simulink model "ALL_JP360_DBW_V6_5_1103"  (R2022a)
settings: Solver=FixedStepAuto  StartTime=0.0  StopTime=inf  FixedStep=0.01  RelTol=1e-3  EnableMultiTasking=on
model workspace (MAT data in the model file):
  g = 9.8
undefined symbols (not defined in the file or in its folder): canChannel, delta_v_p, IPM_Line_C0, IPM_Line_C1, IPM_Line_C2, IPM_Line_C3, M, M_p, MRR_ObjDistX, MRR_ObjDistY, MRR_ObjFusionCamID, MRR_ObjFusionSig, MRR_ObjID, MRR_ObjRelVelX, MRR_ObjRelVelY, MRR_ObjType, MRR_ObjUpdFlg, none, obj_vaild, untracktime, V, videoinput
libraries: canfdmsglib x230, canfdlib x76, slpidlib x24, simulink x18, dspstat3 x14, ctrlSharedLib x1, simulink_extras x1, imaqlib x1, realtime_pacer_lib x1, dspvision x1, visionsinks x1
(part 15 of 55)

== system ALL_JP360_DBW_V6_5_1103/MsgFromCAN/CCAN_GW_MsgFromCAN/CCAN_GW_SRR_FL_0x27B ==
  CCAN_GW_SRR_FL_0x27BFromInData : Inport  OutDataTypeStr=Bus:CAN_FD_MESSAGE_BUS
  Bus Creator : BusCreator  Inputs=8  OutDataTypeStr=Bus:CCAN_GW_SRR_FL_0x27B  NonVirtualBus=on
  CAN FD Unpack : canfdmsglib/CAN FD Unpack  CANdbFile=HiFire_JPT360_CCAN_Matrix_CAN_V1.72_VP_ADCU.dbc  MsgList=(none)  MsgName=SRR_FL_0x27B  ProtocolMode=CAN FD  MsgIDType=Standard (11-bit identifier)  MsgIdentifier=635  MsgLength=8  SignalInfo={'BSD_FCTA_Active','0','2','BE','unsigned','Standard','0','1','0','0','3';'BSD_FCTA_State','7','1','BE','unsigned','Standard','0','1','0','0','1';'BSD_FCTA_display','12','4','BE','unsigned','Standard','0','1','0','0','15';'Checksum_0x27B','56','8','BE','unsigned','Standard','0','1','0','0','255';'FCTA_OFFTelltale','6','1','BE','unsigned','Standard','0','1','0','0','1';'FCTA_warningReqLeft','4','2','BE','unsigned','Standard','0','1','0','0','3';'FCTA_warningReqRight','2','2','BE','unsigned','Standard','0','1','0','0','3';'RollingCounter_0x27B','48','4','BE','unsigned','Standard','0','1','0','0','15'}  IDPort=off  TimestampPort=off  ErrorPort=off  RemotePort=off  LengthPort=off  StatusPort=off  BRSPort=off  ESIPort=off  DLCPort=off  ApplyMinMax=off
      settings: SourceProductBaseCode=XP,ME,VN  DataFormat=CANdb specified signals
  Data Type Conversion{1,3,6..8} (5 alike) : DataTypeConversion  OutDataTypeStr=int8  SaturateOnIntegerOverflow=off  RndMeth=Floor
  Data Type Conversion2 : DataTypeConversion  OutDataTypeStr=boolean  SaturateOnIntegerOverflow=off  RndMeth=Floor
  Data Type Conversion4 : DataTypeConversion  OutDataTypeStr=uint8  SaturateOnIntegerOverflow=off  RndMeth=Floor
  Data Type Conversion5 : DataTypeConversion  OutDataTypeStr=boolean  SaturateOnIntegerOverflow=off  RndMeth=Floor
  CCAN_GW_SRR_FL_0x27BFromOutData : Outport  OutDataTypeStr=Bus:CCAN_GW_SRR_FL_0x27B
  wires:
  CAN FD Unpack/1 -> Data Type Conversion1/1
  CAN FD Unpack/2 -> Data Type Conversion2/1
  CAN FD Unpack/3 -> Data Type Conversion3/1
  CAN FD Unpack/4 -> Data Type Conversion4/1
  CAN FD Unpack/5 -> Data Type Conversion5/1
  CAN FD Unpack/6 -> Data Type Conversion6/1
  CAN FD Unpack/7 -> Data Type Conversion7/1
  CAN FD Unpack/8 -> Data Type Conversion8/1
  Data Type Conversion1/1 -> Bus Creator/1  "BSD_FCTA_Active"
  Data Type Conversion2/1 -> Bus Creator/2  "BSD_FCTA_State"
  Data Type Conversion3/1 -> Bus Creator/3  "BSD_FCTA_display"
  Data Type Conversion4/1 -> Bus Creator/4  "Checksum_0x27B"
  Data Type Conversion5/1 -> Bus Creator/5  "FCTA_OFFTelltale"
  Data Type Conversion6/1 -> Bus Creator/6  "FCTA_warningReqLeft"
  Data Type Conversion7/1 -> Bus Creator/7  "FCTA_warningReqRight"
  Data Type Conversion8/1 -> Bus Creator/8  "RollingCounter_0x27B"
  Bus Creator/1 -> CCAN_GW_SRR_FL_0x27BFromOutData/1  "CCAN_GW_SRR_FL_0x27BFromOutData"
  CCAN_GW_SRR_FL_0x27BFromInData/1 -> CAN FD Unpack/1  "CCAN_GW_SRR_FL_0x27BFromInData"

== system ALL_JP360_DBW_V6_5_1103/MsgFromCAN/CCAN_GW_MsgFromCAN/CCAN_GW_SRR_RL_0x27A ==
  CCAN_GW_SRR_RL_0x27AFromInData : Inport  OutDataTypeStr=Bus:CAN_FD_MESSAGE_BUS
  Bus Creator : BusCreator  Inputs=5  OutDataTypeStr=Bus:CCAN_GW_SRR_RL_0x27A  NonVirtualBus=on
  CAN FD Unpack : canfdmsglib/CAN FD Unpack  CANdbFile=HiFire_JPT360_CCAN_Matrix_CAN_V1.72_VP_ADCU.dbc  MsgList=(none)  MsgName=SRR_RL_0x27A  ProtocolMode=CAN FD  MsgIDType=Standard (11-bit identifier)  MsgIdentifier=634  MsgLength=8  SignalInfo={'BSD_RCTBTargetDeceleration','16','16','BE','unsigned','Standard','0','0.05','-16','-16','16';'BSD_RCTB_State','7','1','BE','unsigned','Standard','0','1','0','0','1';'BSD_RCTB_req','6','1','BE','unsigned','Standard','0','1','0','0','1';'Checksum_0x27A','56','8','BE','unsigned','Standard','0','1','0','0','255';'RollingCounter_0x27A','48','4','BE','unsigned','Standard','0','1','0','0','15'}  IDPort=off  TimestampPort=off  ErrorPort=off  RemotePort=off  LengthPort=off  StatusPort=off  BRSPort=off  ESIPort=off  DLCPort=off  ApplyMinMax=off
      settings: SourceProductBaseCode=XP,ME,VN  DataFormat=CANdb specified signals
  Data Type Conversion1 : DataTypeConversion  OutDataTypeStr=single  SaturateOnIntegerOverflow=off  RndMeth=Floor
  Data Type Conversion2 : DataTypeConversion  OutDataTypeStr=boolean  SaturateOnIntegerOverflow=off  RndMeth=Floor
  Data Type Conversion3 : DataTypeConversion  OutDataTypeStr=boolean  SaturateOnIntegerOverflow=off  RndMeth=Floor
  Data Type Conversion4 : DataTypeConversion  OutDataTypeStr=uint8  SaturateOnIntegerOverflow=off  RndMeth=Floor
  Data Type Conversion5 : DataTypeConversion  OutDataTypeStr=int8  SaturateOnIntegerOverflow=off  RndMeth=Floor
  CCAN_GW_SRR_RL_0x27AFromOutData : Outport  OutDataTypeStr=Bus:CCAN_GW_SRR_RL_0x27A
  wires:
  CAN FD Unpack/1 -> Data Type Conversion1/1
  CAN FD Unpack/2 -> Data Type Conversion2/1
  CAN FD Unpack/3 -> Data Type Conversion3/1
  CAN FD Unpack/4 -> Data Type Conversion4/1
  CAN FD Unpack/5 -> Data Type Conversion5/1
  Data Type Conversion1/1 -> Bus Creator/1  "BSD_RCTBTargetDeceleration"
  Data Type Conversion2/1 -> Bus Creator/2  "BSD_RCTB_State"
  Data Type Conversion3/1 -> Bus Creator/3  "BSD_RCTB_req"
  Data Type Conversion4/1 -> Bus Creator/4  "Checksum_0x27A"
  Data Type Conversion5/1 -> Bus Creator/5  "RollingCounter_0x27A"
  Bus Creator/1 -> CCAN_GW_SRR_RL_0x27AFromOutData/1  "CCAN_GW_SRR_RL_0x27AFromOutData"
  CCAN_GW_SRR_RL_0x27AFromInData/1 -> CAN FD Unpack/1  "CCAN_GW_SRR_RL_0x27AFromInData"

== system ALL_JP360_DBW_V6_5_1103/MsgFromCAN/SRR_ADCU_MsgFromCAN/SRR_ADCU_FLR_AssistSysSt_0x71 ==
  SRR_ADCU_FLR_AssistSysSt_0x71FromInData : Inport  OutDataTypeStr=Bus:CAN_FD_MESSAGE_BUS
  Bus Creator : BusCreator  Inputs=9  OutDataTypeStr=Bus:SRR_ADCU_FLR_AssistSysSt_0x71  NonVirtualBus=on
  CAN FD Unpack : canfdmsglib/CAN FD Unpack  CANdbFile=V363 SRR Private CAN-V1.3.dbc  MsgList=(none)  MsgName=FLR_AssistSysSt_0x71  ProtocolMode=CAN FD  MsgIDType=Standard (11-bit identifier)  MsgIdentifier=113  MsgLength=20  SignalInfo={'CRCCheck_FLR_AssistSysSt','152','16','BE','unsigned','Standard','0','1','0','0','65535';'FLR_Localtime_Nsec','122','30','BE','unsigned','Standard','0','1','0','0','1073741823';'FLR_Localtime_sec','48','32','BE','unsigned','Standard','0','1','0','0','4294967295';'FLR_SRR_Obj_Failure','5','3','BE','unsigned','Standard','0','1','0','0','7';'FLR_SRR_TiBas','63','1','BE','unsigned','Standard','0','1','0','0','1';'FLR_SRR_TiLeap','62','1','BE','unsigned','Standard','0','1','0','0','1';'FLR_SRR_TiOut','61','1','BE','unsigned','Standard','0','1','0','0','1';'FLR_SRR_alignAngle','8','13','BE','unsigned','Standard','0','0.01','0','0','80';'RollingCounter_FLR_AssistSysSt','136','4','BE','unsigned','Standard','0','1','0','0','15'}  IDPort=off  TimestampPort=off  ErrorPort=off  RemotePort=off  LengthPort=off  StatusPort=off  BRSPort=off  ESIPort=off  DLCPort=off  ApplyMinMax=off
      settings: SourceProductBaseCode=ME,XP,VN  DataFormat=CANdb specified signals
  Data Type Conversion1 : DataTypeConversion  OutDataTypeStr=uint16  SaturateOnIntegerOverflow=off  RndMeth=Floor
  Data Type Conversion2 : DataTypeConversion  OutDataTypeStr=int32  SaturateOnIntegerOverflow=off  RndMeth=Floor
  Data Type Conversion3 : DataTypeConversion  OutDataTypeStr=uint32  SaturateOnIntegerOverflow=off  RndMeth=Floor
  Data Type Conversion4 : DataTypeConversion  OutDataTypeStr=int8  SaturateOnIntegerOverflow=off  RndMeth=Floor
  Data Type Conversion5 : DataTypeConversion  OutDataTypeStr=boolean  SaturateOnIntegerOverflow=off  RndMeth=Floor
  Data Type Conversion6 : DataTypeConversion  OutDataTypeStr=boolean  SaturateOnIntegerOverflow=off  RndMeth=Floor
  Data Type Conversion7 : DataTypeConversion  OutDataTypeStr=boolean  SaturateOnIntegerOverflow=off  RndMeth=Floor
  Data Type Conversion8 : DataTypeConversion  OutDataTypeStr=single  SaturateOnIntegerOverflow=off  RndMeth=Floor
  Data Type Conversion9 : DataTypeConversion  OutDataTypeStr=int8  SaturateOnIntegerOverflow=off  RndMeth=Floor
  SRR_ADCU_FLR_AssistSysSt_0x71FromOutData : Outport  OutDataTypeStr=Bus:SRR_ADCU_FLR_AssistSysSt_0x71
  wires:
  CAN FD Unpack/1 -> Data Type Conversion1/1
  CAN FD Unpack/2 -> Data Type Conversion2/1
  CAN FD Unpack/3 -> Data Type Conversion3/1
  CAN FD Unpack/4 -> Data Type Conversion4/1
  CAN FD Unpack/5 -> Data Type Conversion5/1
  CAN FD Unpack/6 -> Data Type Conversion6/1
  CAN FD Unpack/7 -> Data Type Conversion7/1
  CAN FD Unpack/8 -> Data Type Conversion8/1
  CAN FD Unpack/9 -> Data Type Conversion9/1
  Data Type Conversion1/1 -> Bus Creator/1  "CRCCheck_FLR_AssistSysSt"
  Data Type Conversion2/1 -> Bus Creator/2  "FLR_Localtime_Nsec"
  Data Type Conversion3/1 -> Bus Creator/3  "FLR_Localtime_sec"
  Data Type Conversion4/1 -> Bus Creator/4  "FLR_SRR_Obj_Failure"
  Data Type Conversion5/1 -> Bus Creator/5  "FLR_SRR_TiBas"
  Data Type Conversion6/1 -> Bus Creator/6  "FLR_SRR_TiLeap"
  Data Type Conversion7/1 -> Bus Creator/7  "FLR_SRR_TiOut"
  Data Type Conversion8/1 -> Bus Creator/8  "FLR_SRR_alignAngle"
  Data Type Conversion9/1 -> Bus Creator/9  "RollingCounter_FLR_AssistSysSt"
  Bus Creator/1 -> SRR_ADCU_FLR_AssistSysSt_0x71FromOutData/1  "SRR_ADCU_FLR_AssistSysSt_0x71FromOutData"
  SRR_ADCU_FLR_AssistSysSt_0x71FromInData/1 -> CAN FD Unpack/1  "SRR_ADCU_FLR_AssistSysSt_0x71FromInData"

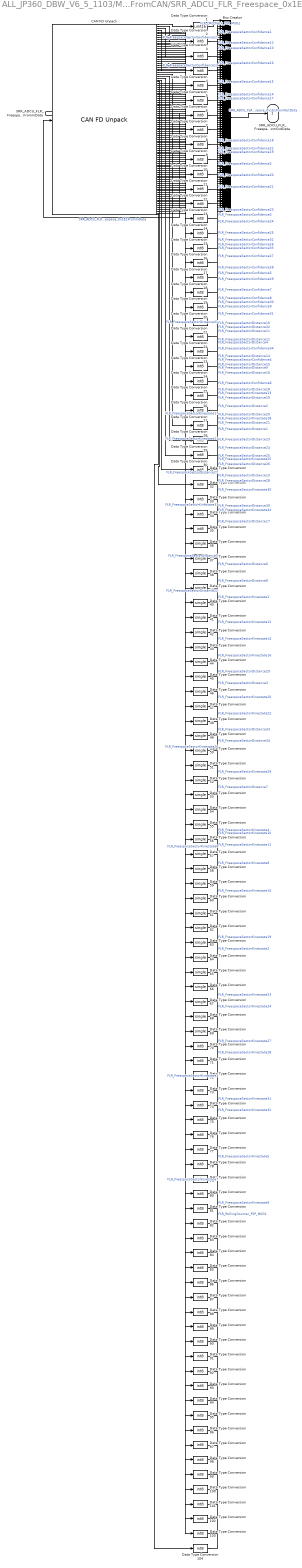
== system ALL_JP360_DBW_V6_5_1103/MsgFromCAN/SRR_ADCU_MsgFromCAN/SRR_ADCU_FLR_Freespace_0x1E1 ==
  SRR_ADCU_FLR_Freespace_0x1E1FromInData : Inport  OutDataTypeStr=Bus:CAN_FD_MESSAGE_BUS
  Bus Creator : BusCreator  Inputs=104  OutDataTypeStr=Bus:SRR_ADCU_FLR_Freespace_0x1E1  NonVirtualBus=on
  CAN FD Unpack : canfdmsglib/CAN FD Unpack  CANdbFile=V363 SRR Private CAN-V1.3.dbc  MsgList=(none)  MsgName=FLR_Freespace_0x1E1  ProtocolMode=CAN FD  MsgIDType=Standard (11-bit identifier)  MsgIdentifier=481  MsgLength=64  SignalInfo={'FLR_CRCCheck_FSP_MSG1','504','16','BE','unsigned','Standard','0','1','0','0','65535';'FLR_FreespaceSectorConfidence1','12','2','BE','unsigned','Standard','0','1','0','0','3';'FLR_FreespaceSectorConfidence10','142','2','BE','unsigned','Standard','0','1','0','0','3';'FLR_FreespaceSectorConfidence11','144','2','BE','unsigned','Standard','0','1','0','0','3';'FLR_FreespaceSectorConfidence12','162','2','BE','unsigned','Standard','0','1','0','0','3';'FLR_FreespaceSectorConfidence13','180','2','BE','unsigned','Standard','0','1','0','0','3';'FLR_FreespaceSectorConfidence14','198','2','BE','unsigned','Standard','0','1','0','0','3';'FLR_FreespaceSectorConfidence15','200','2','BE','unsigned','Standard','0','1','0','0','3';'FLR_FreespaceSectorConfidence16','218','2','BE','unsigned','Standard','0','1','0','0','3';'FLR_FreespaceSectorConfidence17','236','2','BE','unsigned','Standard','0','1','0','0','3';'FLR_FreespaceSectorConfidence18','254','2','BE','unsigned','Standard','0','1','0','0','3';'FLR_FreespaceSectorConfidence19','256','2','BE','unsigned','Standard','0','1','0','0','3';'FLR_FreespaceSectorConfidence2','30','2','BE','unsigned','Standard','0','1','0','0','3';'FLR_FreespaceSectorConfidence20','274','2','BE','unsigned','Standard','0','1','0','0','3';'FLR_FreespaceSectorConfidence21','292','2','BE','unsigned','Standard','0','1','0','0','3';'FLR_FreespaceSectorConfidence22','310','2','BE','unsigned','Standard','0','1','0','0','3';'FLR_FreespaceSectorConfidence23','312','2','BE','unsigned','Standard','0','1','0','0','3';'FLR_FreespaceSectorConfidence24','330','2','BE','unsigned','Standard','0','1','0','0','3';'FLR_FreespaceSectorConfidence25','348','2','BE','unsigned','Standard','0','1','0','0','3';'FLR_FreespaceSectorConfidence26','366','2','BE','unsigned','Standard','0','1','0','0','3';'FLR_FreespaceSectorConfidence27','368','2','BE','unsigned','Standard','0','1','0','0','3';'FLR_FreespaceSectorConfidence28','386','2','BE','unsigned','Standard','0','1','0','0','3';'FLR_FreespaceSectorConfidence29','404','2','BE','unsigned','Standard','0','1','0','0','3';'FLR_FreespaceSectorConfidence3','32','2','BE','unsigned','Standard','0','1','0','0','3';'FLR_FreespaceSectorConfidence30','422','2','BE','unsigned','Standard','0','1','0','0','3';'FLR_FreespaceSectorConfidence31','424','2','BE','unsigned','Standard','0','1','0','0','3';'FLR_FreespaceSectorConfidence32','442','2','BE','unsigned','Standard','0','1','0','0','3';'FLR_FreespaceSectorConfidence33','460','2','BE','unsigned','Standard','0','1','0','0','3';'FLR_FreespaceSectorConfidence34','478','2','BE','unsigned','Standard','0','1','0','0','3';'FLR_FreespaceSectorConfidence4','50','2','BE','unsigned','Standard','0','1','0','0','3';'FLR_FreespaceSectorConfidence5','68','2','BE','unsigned','Standard','0','1','0','0','3';'FLR_FreespaceSectorConfidence6','86','2','BE','unsigned','Standard','0','1','0','0','3';'FLR_FreespaceSectorConfidence7','88','2','BE','unsigned','Standard','0','1','0','0','3';'FLR_FreespaceSectorConfidence8','106','2','BE','unsigned','Standard','0','1','0','0','3';'FLR_FreespaceSectorConfidence9','124','2','BE','unsigned','Standard','0','1','0','0','3';'FLR_FreespaceSectorDistance1','14','10','BE','unsigned','Standard','0','0.1','0','0','100';'FLR_FreespaceSectorDistance10','128','10','BE','unsigned','Standard','0','0.1','0','0','100';'FLR_FreespaceSectorDistance11','146','10','BE','unsigned','Standard','0','0.1','0','0','100';'FLR_FreespaceSectorDistance12','164','10','BE','unsigned','Standard','0','0.1','0','0','100';'FLR_FreespaceSectorDistance13','182','10','BE','unsigned','Standard','0','0.1','0','0','100';'FLR_FreespaceSectorDistance14','184','10','BE','unsigned','Standard','0','0.1','0','0','100';'FLR_FreespaceSectorDistance15','202','10','BE','unsigned','Standard','0','0.1','0','0','100';'FLR_FreespaceSectorDistance16','220','10','BE','unsigned','Standard','0','0.1','0','0','100';'FLR_FreespaceSectorDistance17','238','10','BE','unsigned','Standard','0','0.1','0','0','100';'FLR_FreespaceSectorDistance18','240','10','BE','unsigned','Standard','0','0.1','0','0','100';'FLR_FreespaceSectorDistance19','258','10','BE','unsigned','Standard','0','0.1','0','0','100';'FLR_FreespaceSectorDistance2','16','10','BE','unsigned','Standard','0','0.1','0','0','100';'FLR_FreespaceSectorDistance20','276','10','BE','unsigned','Standard','0','0.1','0','0','100';'FLR_FreespaceSectorDistance21','294','10','BE','unsigned','Standard','0','0.1','0','0','100';'FLR_FreespaceSectorDistance22','296','10','BE','unsigned','Standard','0','0.1','0','0','100';'FLR_FreespaceSectorDistance23','314','10','BE','unsigned','Standard','0','0.1','0','0','100';'FLR_FreespaceSectorDistance24','332','10','BE','unsigned','Standard','0','0.1','0','0','100';'FLR_FreespaceSectorDistance25','350','10','BE','unsigned','Standard','0','0.1','0','0','100';'FLR_FreespaceSectorDistance26','352','10','BE','unsigned','Standard','0','0.1','0','0','100';'FLR_FreespaceSectorDistance27','370','10','BE','unsigned','Standard','0','0.1','0','0','100';'FLR_FreespaceSectorDistance28','388','10','BE','unsigned','Standard','0','0.1','0','0','100';'FLR_FreespaceSectorDistance29','406','10','BE','unsigned','Standard','0','0.1','0','0','100';'FLR_FreespaceSectorDistance3','34','10','BE','unsigned','Standard','0','0.1','0','0','100';'FLR_FreespaceSectorDistance30','408','10','BE','unsigned','Standard','0','0.1','0','0','100';'FLR_FreespaceSectorDistance31','426','10','BE','unsigned','Standard','0','0.1','0','0','100';'FLR_FreespaceSectorDistance32','444','10','BE','unsigned','Standard','0','0.1','0','0','100';'FLR_FreespaceSectorDistance33','462','10','BE','unsigned','Standard','0','0.1','0','0','100';'FLR_FreespaceSectorDistance34','464','10','BE','unsigned','Standard','0','0.1','0','0','100';'FLR_FreespaceSectorDistance4','52','10','BE','unsigned','Standard','0','0.1','0','0','100';'FLR_FreespaceSectorDistance5','70','10','BE','unsigned','Standard','0','0.1','0','0','100';'FLR_FreespaceSectorDistance6','72','10','BE','unsigned','Standard','0','0.1','0','0','100';'FLR_FreespaceSectorDistance7','90','10','BE','unsigned','Standard','0','0.1','0','0','100';'FLR_FreespaceSectorDistance8','108','10','BE','unsigned','Standard','0','0.1','0','0','100';'FLR_FreespaceSectorDistance9','126','10','BE','unsigned','Standard','0','0.1','0','0','100';'FLR_FreespaceSectorKinestate1','10','2','BE','unsigned','Standard','0','1','0','0','3';'FLR_FreespaceSectorKinestate10','140','2','BE','unsigned','Standard','0','1','0','0','3';'FLR_FreespaceSectorKinestate11','158','2','BE','unsigned','Standard','0','1','0','0','3';'FLR_FreespaceSectorKinestate12','160','2','BE','unsigned','Standard','0','1','0','0','3';'FLR_FreespaceSectorKinestate13','178','2','BE','unsigned','Standard','0','1','0','0','3';'FLR_FreespaceSectorKinestate14','196','2','BE','unsigned','Standard','0','1','0','0','3';'FLR_FreespaceSectorKinestate15','214','2','BE','unsigned','Standard','0','1','0','0','3';'FLR_FreespaceSectorKinestate16','216','2','BE','unsigned','Standard','0','1','0','0','3';'FLR_FreespaceSectorKinestate17','234','2','BE','unsigned','Standard','0','1','0','0','3';'FLR_FreespaceSectorKinestate18','252','2','BE','unsigned','Standard','0','1','0','0','3';'FLR_FreespaceSectorKinestate19','270','2','BE','unsigned','Standard','0','1','0','0','3';'FLR_FreespaceSectorKinestate2','28','2','BE','unsigned','Standard','0','1','0','0','3';'FLR_FreespaceSectorKinestate20','272','2','BE','unsigned','Standard','0','1','0','0','3';'FLR_FreespaceSectorKinestate21','290','2','BE','unsigned','Standard','0','1','0','0','3';'FLR_FreespaceSectorKinestate22','308','2','BE','unsigned','Standard','0','1','0','0','3';'FLR_FreespaceSectorKinestate23','326','2','BE','unsigned','Standard','0','1','0','0','3';'FLR_FreespaceSectorKinestate24','328','2','BE','unsigned','Standard','0','1','0','0','3';'FLR_FreespaceSectorKinestate25','346','2','BE','unsigned','Standard','0','1','0','0','3';'FLR_FreespaceSectorKinestate26','364','2','BE','unsigned','Standard','0','1','0','0','3';'FLR_FreespaceSectorKinestate27','382','2','BE','unsigned','Standard','0','1','0','0','3';'FLR_FreespaceSectorKinestate28','384','2','BE','unsigned','Standard','0','1','0','0','3';'FLR_FreespaceSectorKinestate29','402','2','BE','unsigned','Standard','0','1','0','0','3';'FLR_FreespaceSectorKinestate3','46','2','BE','unsigned','Standard','0','1','0','0','3';'FLR_FreespaceSectorKinestate30','420','2','BE','unsigned','Standard','0','1','0','0','3';'FLR_FreespaceSectorKinestate31','438','2','BE','unsigned','Standard','0','1','0','0','3';'FLR_FreespaceSectorKinestate32','440','2','BE','unsigned','Standard','0','1','0','0','3';'FLR_FreespaceSectorKinestate33','458','2','BE','unsigned','Standard','0','1','0','0','3';'FLR_FreespaceSectorKinestate34','476','2','BE','unsigned','Standard','0','1','0','0','3';'FLR_FreespaceSectorKinestate4','48','2','BE','unsigned','Standard','0','1','0','0','3';'FLR_FreespaceSectorKinestate5','66','2','BE','unsigned','Standard','0','1','0','0','3';'FLR_FreespaceSectorKinestate6','84','2','BE','unsigned','Standard','0','1','0','0','3';'FLR_FreespaceSectorKinestate7','102','2','BE','unsigned','Standard','0','1','0','0','3';'FLR_FreespaceSectorKinestate8','104','2','BE','unsigned','Standard','0','1','0','0','3';'FLR_FreespaceSectorKinestate9','122','2','BE','unsigned','Standard','0','1','0','0','3';'FLR_RollingCounter_FSP_MSG1','488','4','BE','unsigned','Standard','0','1','0','0','15'}  IDPort=off  TimestampPort=off  ErrorPort=off  RemotePort=off  LengthPort=off  StatusPort=off  BRSPort=off  ESIPort=off  DLCPort=off  ApplyMinMax=off
      settings: SourceProductBaseCode=ME,XP,VN  DataFormat=CANdb specified signals
  Data Type Conversion1 : DataTypeConversion  OutDataTypeStr=uint16  SaturateOnIntegerOverflow=off  RndMeth=Floor
  Data Type Conversion{2..35,70..104} (69 alike) : DataTypeConversion  OutDataTypeStr=int8  SaturateOnIntegerOverflow=off  RndMeth=Floor
  Data Type Conversion{36..69} (34 alike) : DataTypeConversion  OutDataTypeStr=single  SaturateOnIntegerOverflow=off  RndMeth=Floor
  SRR_ADCU_FLR_Freespace_0x1E1FromOutData : Outport  OutDataTypeStr=Bus:SRR_ADCU_FLR_Freespace_0x1E1
  wires:
  CAN FD Unpack/1 -> Data Type Conversion1/1
  CAN FD Unpack/2 -> Data Type Conversion2/1
  CAN FD Unpack/3 -> Data Type Conversion3/1
  CAN FD Unpack/4 -> Data Type Conversion4/1
  CAN FD Unpack/5 -> Data Type Conversion5/1
  CAN FD Unpack/6 -> Data Type Conversion6/1
  CAN FD Unpack/7 -> Data Type Conversion7/1
  CAN FD Unpack/8 -> Data Type Conversion8/1
  CAN FD Unpack/9 -> Data Type Conversion9/1
  CAN FD Unpack/10 -> Data Type Conversion10/1
  CAN FD Unpack/11 -> Data Type Conversion11/1
  CAN FD Unpack/12 -> Data Type Conversion12/1
  CAN FD Unpack/13 -> Data Type Conversion13/1
  CAN FD Unpack/14 -> Data Type Conversion14/1
  CAN FD Unpack/15 -> Data Type Conversion15/1
  CAN FD Unpack/16 -> Data Type Conversion16/1
  CAN FD Unpack/17 -> Data Type Conversion17/1
  CAN FD Unpack/18 -> Data Type Conversion18/1
  CAN FD Unpack/19 -> Data Type Conversion19/1
  CAN FD Unpack/20 -> Data Type Conversion20/1
  CAN FD Unpack/21 -> Data Type Conversion21/1
  CAN FD Unpack/22 -> Data Type Conversion22/1
  CAN FD Unpack/23 -> Data Type Conversion23/1
  CAN FD Unpack/24 -> Data Type Conversion24/1
  CAN FD Unpack/25 -> Data Type Conversion25/1
  CAN FD Unpack/26 -> Data Type Conversion26/1
  CAN FD Unpack/27 -> Data Type Conversion27/1
  CAN FD Unpack/28 -> Data Type Conversion28/1
  CAN FD Unpack/29 -> Data Type Conversion29/1
  CAN FD Unpack/30 -> Data Type Conversion30/1
  CAN FD Unpack/31 -> Data Type Conversion31/1
  CAN FD Unpack/32 -> Data Type Conversion32/1
  CAN FD Unpack/33 -> Data Type Conversion33/1
  CAN FD Unpack/34 -> Data Type Conversion34/1
  CAN FD Unpack/35 -> Data Type Conversion35/1
  CAN FD Unpack/36 -> Data Type Conversion36/1
  CAN FD Unpack/37 -> Data Type Conversion37/1
  CAN FD Unpack/38 -> Data Type Conversion38/1
  CAN FD Unpack/39 -> Data Type Conversion39/1
  CAN FD Unpack/40 -> Data Type Conversion40/1
  CAN FD Unpack/41 -> Data Type Conversion41/1
  CAN FD Unpack/42 -> Data Type Conversion42/1
  CAN FD Unpack/43 -> Data Type Conversion43/1
  CAN FD Unpack/44 -> Data Type Conversion44/1
  CAN FD Unpack/45 -> Data Type Conversion45/1
  CAN FD Unpack/46 -> Data Type Conversion46/1
  CAN FD Unpack/47 -> Data Type Conversion47/1
  CAN FD Unpack/48 -> Data Type Conversion48/1
  CAN FD Unpack/49 -> Data Type Conversion49/1
  CAN FD Unpack/50 -> Data Type Conversion50/1
  CAN FD Unpack/51 -> Data Type Conversion51/1
  CAN FD Unpack/52 -> Data Type Conversion52/1
  CAN FD Unpack/53 -> Data Type Conversion53/1
  CAN FD Unpack/54 -> Data Type Conversion54/1
  CAN FD Unpack/55 -> Data Type Conversion55/1
  CAN FD Unpack/56 -> Data Type Conversion56/1
  CAN FD Unpack/57 -> Data Type Conversion57/1
  CAN FD Unpack/58 -> Data Type Conversion58/1
  CAN FD Unpack/59 -> Data Type Conversion59/1
  CAN FD Unpack/60 -> Data Type Conversion60/1
  CAN FD Unpack/61 -> Data Type Conversion61/1
  CAN FD Unpack/62 -> Data Type Conversion62/1
  CAN FD Unpack/63 -> Data Type Conversion63/1
  CAN FD Unpack/64 -> Data Type Conversion64/1
  CAN FD Unpack/65 -> Data Type Conversion65/1
  CAN FD Unpack/66 -> Data Type Conversion66/1
  CAN FD Unpack/67 -> Data Type Conversion67/1
  CAN FD Unpack/68 -> Data Type Conversion68/1
  CAN FD Unpack/69 -> Data Type Conversion69/1
  CAN FD Unpack/70 -> Data Type Conversion70/1
  CAN FD Unpack/71 -> Data Type Conversion71/1
  CAN FD Unpack/72 -> Data Type Conversion72/1
  CAN FD Unpack/73 -> Data Type Conversion73/1
  CAN FD Unpack/74 -> Data Type Conversion74/1
  CAN FD Unpack/75 -> Data Type Conversion75/1
  CAN FD Unpack/76 -> Data Type Conversion76/1
  CAN FD Unpack/77 -> Data Type Conversion77/1
  CAN FD Unpack/78 -> Data Type Conversion78/1
  CAN FD Unpack/79 -> Data Type Conversion79/1
  CAN FD Unpack/80 -> Data Type Conversion80/1
  CAN FD Unpack/81 -> Data Type Conversion81/1
  CAN FD Unpack/82 -> Data Type Conversion82/1
  CAN FD Unpack/83 -> Data Type Conversion83/1
  CAN FD Unpack/84 -> Data Type Conversion84/1
  CAN FD Unpack/85 -> Data Type Conversion85/1
  CAN FD Unpack/86 -> Data Type Conversion86/1
  CAN FD Unpack/87 -> Data Type Conversion87/1
  CAN FD Unpack/88 -> Data Type Conversion88/1
  CAN FD Unpack/89 -> Data Type Conversion89/1
  CAN FD Unpack/90 -> Data Type Conversion90/1
  CAN FD Unpack/91 -> Data Type Conversion91/1
  CAN FD Unpack/92 -> Data Type Conversion92/1
  CAN FD Unpack/93 -> Data Type Conversion93/1
  CAN FD Unpack/94 -> Data Type Conversion94/1
  CAN FD Unpack/95 -> Data Type Conversion95/1
  CAN FD Unpack/96 -> Data Type Conversion96/1
  CAN FD Unpack/97 -> Data Type Conversion97/1
  CAN FD Unpack/98 -> Data Type Conversion98/1
  CAN FD Unpack/99 -> Data Type Conversion99/1
  CAN FD Unpack/100 -> Data Type Conversion100/1
  CAN FD Unpack/101 -> Data Type Conversion101/1
  CAN FD Unpack/102 -> Data Type Conversion102/1
  CAN FD Unpack/103 -> Data Type Conversion103/1
  CAN FD Unpack/104 -> Data Type Conversion104/1
  Data Type Conversion1/1 -> Bus Creator/1  "FLR_CRCCheck_FSP_MSG1"
  Data Type Conversion2/1 -> Bus Creator/2  "FLR_FreespaceSectorConfidence1"
  Data Type Conversion3/1 -> Bus Creator/3  "FLR_FreespaceSectorConfidence10"
  Data Type Conversion4/1 -> Bus Creator/4  "FLR_FreespaceSectorConfidence11"
  Data Type Conversion5/1 -> Bus Creator/5  "FLR_FreespaceSectorConfidence12"
  Data Type Conversion6/1 -> Bus Creator/6  "FLR_FreespaceSectorConfidence13"
  Data Type Conversion7/1 -> Bus Creator/7  "FLR_FreespaceSectorConfidence14"
  Data Type Conversion8/1 -> Bus Creator/8  "FLR_FreespaceSectorConfidence15"
  Data Type Conversion9/1 -> Bus Creator/9  "FLR_FreespaceSectorConfidence16"
  Data Type Conversion10/1 -> Bus Creator/10  "FLR_FreespaceSectorConfidence17"
  Data Type Conversion11/1 -> Bus Creator/11  "FLR_FreespaceSectorConfidence18"
  Data Type Conversion12/1 -> Bus Creator/12  "FLR_FreespaceSectorConfidence19"
  Data Type Conversion13/1 -> Bus Creator/13  "FLR_FreespaceSectorConfidence2"
  Data Type Conversion14/1 -> Bus Creator/14  "FLR_FreespaceSectorConfidence20"
  Data Type Conversion15/1 -> Bus Creator/15  "FLR_FreespaceSectorConfidence21"
  Data Type Conversion16/1 -> Bus Creator/16  "FLR_FreespaceSectorConfidence22"
  Data Type Conversion17/1 -> Bus Creator/17  "FLR_FreespaceSectorConfidence23"
  Data Type Conversion18/1 -> Bus Creator/18  "FLR_FreespaceSectorConfidence24"
  Data Type Conversion19/1 -> Bus Creator/19  "FLR_FreespaceSectorConfidence25"
  Data Type Conversion20/1 -> Bus Creator/20  "FLR_FreespaceSectorConfidence26"
  Data Type Conversion21/1 -> Bus Creator/21  "FLR_FreespaceSectorConfidence27"
  Data Type Conversion22/1 -> Bus Creator/22  "FLR_FreespaceSectorConfidence28"
  Data Type Conversion23/1 -> Bus Creator/23  "FLR_FreespaceSectorConfidence29"
  Data Type Conversion24/1 -> Bus Creator/24  "FLR_FreespaceSectorConfidence3"
  Data Type Conversion25/1 -> Bus Creator/25  "FLR_FreespaceSectorConfidence30"
  Data Type Conversion26/1 -> Bus Creator/26  "FLR_FreespaceSectorConfidence31"
  Data Type Conversion27/1 -> Bus Creator/27  "FLR_FreespaceSectorConfidence32"
  Data Type Conversion28/1 -> Bus Creator/28  "FLR_FreespaceSectorConfidence33"
  Data Type Conversion29/1 -> Bus Creator/29  "FLR_FreespaceSectorConfidence34"
  Data Type Conversion30/1 -> Bus Creator/30  "FLR_FreespaceSectorConfidence4"
  Data Type Conversion31/1 -> Bus Creator/31  "FLR_FreespaceSectorConfidence5"
  Data Type Conversion32/1 -> Bus Creator/32  "FLR_FreespaceSectorConfidence6"
  Data Type Conversion33/1 -> Bus Creator/33  "FLR_FreespaceSectorConfidence7"
  Data Type Conversion34/1 -> Bus Creator/34  "FLR_FreespaceSectorConfidence8"
  Data Type Conversion35/1 -> Bus Creator/35  "FLR_FreespaceSectorConfidence9"
  Data Type Conversion36/1 -> Bus Creator/36  "FLR_FreespaceSectorDistance1"
  Data Type Conversion37/1 -> Bus Creator/37  "FLR_FreespaceSectorDistance10"
  Data Type Conversion38/1 -> Bus Creator/38  "FLR_FreespaceSectorDistance11"
  Data Type Conversion39/1 -> Bus Creator/39  "FLR_FreespaceSectorDistance12"
  Data Type Conversion40/1 -> Bus Creator/40  "FLR_FreespaceSectorDistance13"
  Data Type Conversion41/1 -> Bus Creator/41  "FLR_FreespaceSectorDistance14"
  Data Type Conversion42/1 -> Bus Creator/42  "FLR_FreespaceSectorDistance15"
  Data Type Conversion43/1 -> Bus Creator/43  "FLR_FreespaceSectorDistance16"
  Data Type Conversion44/1 -> Bus Creator/44  "FLR_FreespaceSectorDistance17"
  Data Type Conversion45/1 -> Bus Creator/45  "FLR_FreespaceSectorDistance18"
  Data Type Conversion46/1 -> Bus Creator/46  "FLR_FreespaceSectorDistance19"
  Data Type Conversion47/1 -> Bus Creator/47  "FLR_FreespaceSectorDistance2"
  Data Type Conversion48/1 -> Bus Creator/48  "FLR_FreespaceSectorDistance20"
  Data Type Conversion49/1 -> Bus Creator/49  "FLR_FreespaceSectorDistance21"
  Data Type Conversion50/1 -> Bus Creator/50  "FLR_FreespaceSectorDistance22"
  Data Type Conversion51/1 -> Bus Creator/51  "FLR_FreespaceSectorDistance23"
  Data Type Conversion52/1 -> Bus Creator/52  "FLR_FreespaceSectorDistance24"
  Data Type Conversion53/1 -> Bus Creator/53  "FLR_FreespaceSectorDistance25"
  Data Type Conversion54/1 -> Bus Creator/54  "FLR_FreespaceSectorDistance26"
  Data Type Conversion55/1 -> Bus Creator/55  "FLR_FreespaceSectorDistance27"
  Data Type Conversion56/1 -> Bus Creator/56  "FLR_FreespaceSectorDistance28"
  Data Type Conversion57/1 -> Bus Creator/57  "FLR_FreespaceSectorDistance29"
  Data Type Conversion58/1 -> Bus Creator/58  "FLR_FreespaceSectorDistance3"
  Data Type Conversion59/1 -> Bus Creator/59  "FLR_FreespaceSectorDistance30"
  Data Type Conversion60/1 -> Bus Creator/60  "FLR_FreespaceSectorDistance31"
  Data Type Conversion61/1 -> Bus Creator/61  "FLR_FreespaceSectorDistance32"
  Data Type Conversion62/1 -> Bus Creator/62  "FLR_FreespaceSectorDistance33"
  Data Type Conversion63/1 -> Bus Creator/63  "FLR_FreespaceSectorDistance34"
  Data Type Conversion64/1 -> Bus Creator/64  "FLR_FreespaceSectorDistance4"
  Data Type Conversion65/1 -> Bus Creator/65  "FLR_FreespaceSectorDistance5"
  Data Type Conversion66/1 -> Bus Creator/66  "FLR_FreespaceSectorDistance6"
  Data Type Conversion67/1 -> Bus Creator/67  "FLR_FreespaceSectorDistance7"
  Data Type Conversion68/1 -> Bus Creator/68  "FLR_FreespaceSectorDistance8"
  Data Type Conversion69/1 -> Bus Creator/69  "FLR_FreespaceSectorDistance9"
  Data Type Conversion70/1 -> Bus Creator/70  "FLR_FreespaceSectorKinestate1"
  Data Type Conversion71/1 -> Bus Creator/71  "FLR_FreespaceSectorKinestate10"
  Data Type Conversion72/1 -> Bus Creator/72  "FLR_FreespaceSectorKinestate11"
  Data Type Conversion73/1 -> Bus Creator/73  "FLR_FreespaceSectorKinestate12"
  Data Type Conversion74/1 -> Bus Creator/74  "FLR_FreespaceSectorKinestate13"
  Data Type Conversion75/1 -> Bus Creator/75  "FLR_FreespaceSectorKinestate14"
  Data Type Conversion76/1 -> Bus Creator/76  "FLR_FreespaceSectorKinestate15"
  Data Type Conversion77/1 -> Bus Creator/77  "FLR_FreespaceSectorKinestate16"
  Data Type Conversion78/1 -> Bus Creator/78  "FLR_FreespaceSectorKinestate17"
  Data Type Conversion79/1 -> Bus Creator/79  "FLR_FreespaceSectorKinestate18"
  Data Type Conversion80/1 -> Bus Creator/80  "FLR_FreespaceSectorKinestate19"
  Data Type Conversion81/1 -> Bus Creator/81  "FLR_FreespaceSectorKinestate2"
  Data Type Conversion82/1 -> Bus Creator/82  "FLR_FreespaceSectorKinestate20"
  Data Type Conversion83/1 -> Bus Creator/83  "FLR_FreespaceSectorKinestate21"
  Data Type Conversion84/1 -> Bus Creator/84  "FLR_FreespaceSectorKinestate22"
  Data Type Conversion85/1 -> Bus Creator/85  "FLR_FreespaceSectorKinestate23"
  Data Type Conversion86/1 -> Bus Creator/86  "FLR_FreespaceSectorKinestate24"
  Data Type Conversion87/1 -> Bus Creator/87  "FLR_FreespaceSectorKinestate25"
  Data Type Conversion88/1 -> Bus Creator/88  "FLR_FreespaceSectorKinestate26"
  Data Type Conversion89/1 -> Bus Creator/89  "FLR_FreespaceSectorKinestate27"
  Data Type Conversion90/1 -> Bus Creator/90  "FLR_FreespaceSectorKinestate28"
  Data Type Conversion91/1 -> Bus Creator/91  "FLR_FreespaceSectorKinestate29"
  Data Type Conversion92/1 -> Bus Creator/92  "FLR_FreespaceSectorKinestate3"
  Data Type Conversion93/1 -> Bus Creator/93  "FLR_FreespaceSectorKinestate30"
  Data Type Conversion94/1 -> Bus Creator/94  "FLR_FreespaceSectorKinestate31"
  Data Type Conversion95/1 -> Bus Creator/95  "FLR_FreespaceSectorKinestate32"
  Data Type Conversion96/1 -> Bus Creator/96  "FLR_FreespaceSectorKinestate33"
  Data Type Conversion97/1 -> Bus Creator/97  "FLR_FreespaceSectorKinestate34"
  Data Type Conversion98/1 -> Bus Creator/98  "FLR_FreespaceSectorKinestate4"
  Data Type Conversion99/1 -> Bus Creator/99  "FLR_FreespaceSectorKinestate5"
  Data Type Conversion100/1 -> Bus Creator/100  "FLR_FreespaceSectorKinestate6"
  Data Type Conversion101/1 -> Bus Creator/101  "FLR_FreespaceSectorKinestate7"
  Data Type Conversion102/1 -> Bus Creator/102  "FLR_FreespaceSectorKinestate8"
  Data Type Conversion103/1 -> Bus Creator/103  "FLR_FreespaceSectorKinestate9"
  Data Type Conversion104/1 -> Bus Creator/104  "FLR_RollingCounter_FSP_MSG1"
  Bus Creator/1 -> SRR_ADCU_FLR_Freespace_0x1E1FromOutData/1  "SRR_ADCU_FLR_Freespace_0x1E1FromOutData"
  SRR_ADCU_FLR_Freespace_0x1E1FromInData/1 -> CAN FD Unpack/1  "SRR_ADCU_FLR_Freespace_0x1E1FromInData"
